simulink library "TYPEB_MASTER"  (Simulink 8.8)
settings: Solver=ode45  StartTime=0.0  StopTime=10.0  RelTol=1e-3  EnableMultiTasking=on
libraries: cdsEpicsOut x65, cdsTP x48, cdsFilt x34, cdsEpicsStringIn x29, cdsFiltCtrl x27, cdsRms x24, STATE_BIO_MASTER x15, cdsEpicsBinIn x14, cdsBit2Word x12, GAS_MASTER x9, cdsWord2Bit x5, cdsDacKill x4
(part 1 of 6)
settings Model: SuppressorTable=22 serialization::archive 11 0 3 0 0 0 11 0  Creator=controls  LastModifiedBy=controls

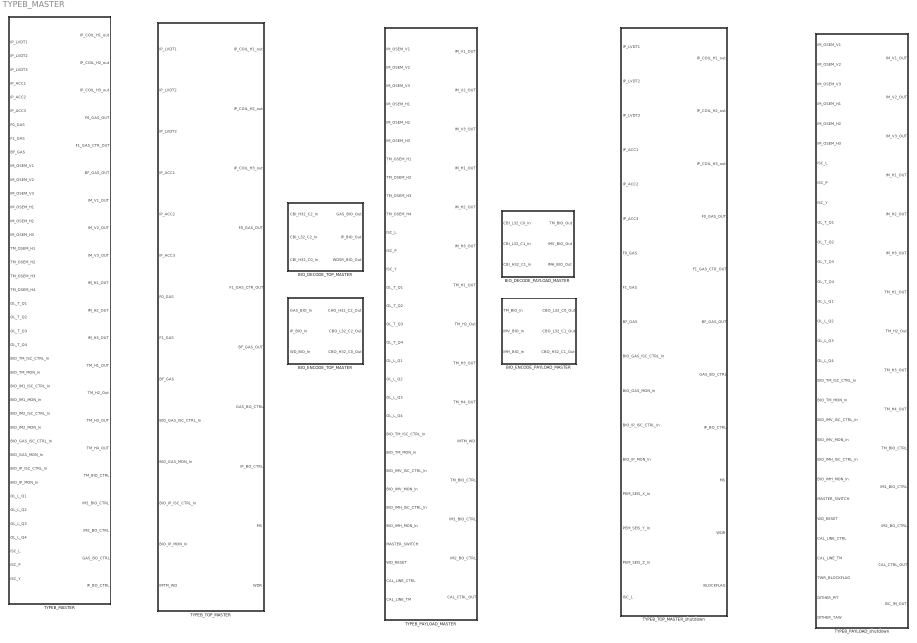
== system TYPEB_MASTER ==
  BIO_DECODE_PAYLOAD_MASTER : Subsystem
  BIO_DECODE_TOP_MASTER : Subsystem
  BIO_ENCODE_PAYLOAD_MASTER : Subsystem
  BIO_ENCODE_TOP_MASTER : Subsystem
  TYPEB_MASTER : Subsystem
  TYPEB_PAYLOAD_MASTER : Subsystem
  TYPEB_PAYLOAD_shutdown : Subsystem  AncestorBlock=TYPEB_MASTER/TYPEB_PAYLOAD_MASTER
  TYPEB_TOP_MASTER : Subsystem
  TYPEB_TOP_MASTER_shutdown : Subsystem  AncestorBlock=TYPEB_MASTER/TYPEB_TOP_MASTER

== system TYPEB_MASTER/BIO_DECODE_PAYLOAD_MASTER ==
  CBI_L32_C0_In : Inport
  CBI_L32_C1_In : Inport  Port=2
  CBI_H32_C1_In : Inport  Port=3
  BI0L_MON : cdsEpicsOut/Subsystem  Tag=cdsEpicsOutput  Description=|
      | Purpose:                                          
      | Output a FE signal to an EPICS channel.           
      |                                                   
      | Operation:                                        
      | Takes input value and passes it to EPICS record.  
      |                                                   
      | Usage:                                            
      | Name the part with the desired EPICS rrecord name.
      settings: AttributesFormatString=%<Tag>
  BI1H_MON : cdsEpicsOut/Subsystem  Tag=cdsEpicsOutput  Description=|
      | Purpose:                                          
      | Output a FE signal to an EPICS channel.           
      |                                                   
      | Operation:                                        
      | Takes input value and passes it to EPICS record.  
      |                                                   
      | Usage:                                            
      | Name the part with the desired EPICS rrecord name.
      settings: AttributesFormatString=%<Tag>
  BI1L_MON : cdsEpicsOut/Subsystem  Tag=cdsEpicsOutput  Description=|
      | Purpose:                                          
      | Output a FE signal to an EPICS channel.           
      |                                                   
      | Operation:                                        
      | Takes input value and passes it to EPICS record.  
      |                                                   
      | Usage:                                            
      | Name the part with the desired EPICS rrecord name.
      settings: AttributesFormatString=%<Tag>
  TM_BIO_Out : Outport
  IMV_BIO_Out : Outport  Port=2
  IMH_BIO_Out : Outport  Port=3
  wires:
  CBI_L32_C1_In/1 -> BI1L_MON/1
  CBI_L32_C0_In/1 -> BI0L_MON/1
  CBI_H32_C1_In/1 -> BI1H_MON/1
  BI0L_MON/1 -> TM_BIO_Out/1
  BI1L_MON/1 -> IMV_BIO_Out/1
  BI1H_MON/1 -> IMH_BIO_Out/1

== system TYPEB_MASTER/BIO_DECODE_TOP_MASTER ==
  CBI_H32_C2_In : Inport
  CBI_L32_C2_In : Inport  Port=2
  CBI_H32_C0_In : Inport  Port=3
  BI0H_MON : cdsEpicsOut/Subsystem  Tag=cdsEpicsOutput  Description=|
      | Purpose:                                          
      | Output a FE signal to an EPICS channel.           
      |                                                   
      | Operation:                                        
      | Takes input value and passes it to EPICS record.  
      |                                                   
      | Usage:                                            
      | Name the part with the desired EPICS rrecord name.
      settings: AttributesFormatString=%<Tag>
  BI2H_MON : cdsEpicsOut/Subsystem  Tag=cdsEpicsOutput  Description=|
      | Purpose:                                          
      | Output a FE signal to an EPICS channel.           
      |                                                   
      | Operation:                                        
      | Takes input value and passes it to EPICS record.  
      |                                                   
      | Usage:                                            
      | Name the part with the desired EPICS rrecord name.
      settings: AttributesFormatString=%<Tag>
  BI2L_MON : cdsEpicsOut/Subsystem  Tag=cdsEpicsOutput  Description=|
      | Purpose:                                          
      | Output a FE signal to an EPICS channel.           
      |                                                   
      | Operation:                                        
      | Takes input value and passes it to EPICS record.  
      |                                                   
      | Usage:                                            
      | Name the part with the desired EPICS rrecord name.
      settings: AttributesFormatString=%<Tag>
  GAS_BIO_Out : Outport
  IP_BIO_Out : Outport  Port=2
  WDSR_BIO_Out : Outport  Port=3
  wires:
  CBI_H32_C2_In/1 -> BI2H_MON/1
  CBI_L32_C2_In/1 -> BI2L_MON/1
  BI2H_MON/1 -> GAS_BIO_Out/1
  BI2L_MON/1 -> IP_BIO_Out/1
  CBI_H32_C0_In/1 -> BI0H_MON/1
  BI0H_MON/1 -> WDSR_BIO_Out/1

== system TYPEB_MASTER/BIO_ENCODE_PAYLOAD_MASTER ==
  TM_BIO_In : Inport
  IMV_BIO_In : Inport  Port=2
  IMH_BIO_In : Inport  Port=3
  BIT2WORD2 : Subsystem
  BIT2WORD3 : Subsystem
  BIT2WORD4 : Subsystem
  BO0L_OUT : cdsEpicsOut/Subsystem  Tag=cdsEpicsOutput  Description=|
      | Purpose:                                          
      | Output a FE signal to an EPICS channel.           
      |                                                   
      | Operation:                                        
      | Takes input value and passes it to EPICS record.  
      |                                                   
      | Usage:                                            
      | Name the part with the desired EPICS rrecord name.
      settings: AttributesFormatString=%<Tag>
  BO1H_OUT : cdsEpicsOut/Subsystem  Tag=cdsEpicsOutput  Description=|
      | Purpose:                                          
      | Output a FE signal to an EPICS channel.           
      |                                                   
      | Operation:                                        
      | Takes input value and passes it to EPICS record.  
      |                                                   
      | Usage:                                            
      | Name the part with the desired EPICS rrecord name.
      settings: AttributesFormatString=%<Tag>
  BO1L_OUT : cdsEpicsOut/Subsystem  Tag=cdsEpicsOutput  Description=|
      | Purpose:                                          
      | Output a FE signal to an EPICS channel.           
      |                                                   
      | Operation:                                        
      | Takes input value and passes it to EPICS record.  
      |                                                   
      | Usage:                                            
      | Name the part with the desired EPICS rrecord name.
      settings: AttributesFormatString=%<Tag>
  Ground{1..3,26,66..67} (6 alike) : Ground
  IMH_WD_RSET : cdsEpicsBinIn/Subsystem  Tag=cdsEpicsBinIn  Description=|
      | Purpose:                                                                            
      | Create an EPICS binary (0 or 1) input channel to the FE realtime controls.          
      |                                                                                     
      | Operation:                                                                          
      | Outputs value from an EPICS ai record. Value is binary input (bi Epics record type).
      |                                                                                     
      | Usage:                                                                              
      | Name the part with the desired EPICS channel name.
      settings: AttributesFormatString=%<Tag>
  IMV_WD_RSET : cdsEpicsBinIn/Subsystem  Tag=cdsEpicsBinIn  Description=|
      | Purpose:                                                                            
      | Create an EPICS binary (0 or 1) input channel to the FE realtime controls.          
      |                                                                                     
      | Operation:                                                                          
      | Outputs value from an EPICS ai record. Value is binary input (bi Epics record type).
      |                                                                                     
      | Usage:                                                                              
      | Name the part with the desired EPICS channel name.
      settings: AttributesFormatString=%<Tag>
  TM_WD_RSET : cdsEpicsBinIn/Subsystem  Tag=cdsEpicsBinIn  Description=|
      | Purpose:                                                                            
      | Create an EPICS binary (0 or 1) input channel to the FE realtime controls.          
      |                                                                                     
      | Operation:                                                                          
      | Outputs value from an EPICS ai record. Value is binary input (bi Epics record type).
      |                                                                                     
      | Usage:                                                                              
      | Name the part with the desired EPICS channel name.
      settings: AttributesFormatString=%<Tag>
  cdsWord2Bit : cdsWord2Bit/cdsWord2Bit  Tag=cdsWord2Bit  Description=Generate 16 0/1 outputs from single 16-bit integer input
      settings: AttributesFormatString=cdsWord2Bit
  cdsWord2Bit1 : cdsWord2Bit/cdsWord2Bit  Tag=cdsWord2Bit  Description=Generate 16 0/1 outputs from single 16-bit integer input
      settings: AttributesFormatString=cdsWord2Bit
  cdsWord2Bit2 : cdsWord2Bit/cdsWord2Bit  Tag=cdsWord2Bit  Description=Generate 16 0/1 outputs from single 16-bit integer input
      settings: AttributesFormatString=cdsWord2Bit
  CBO_L32_C0_Out : Outport
  CBO_L32_C1_Out : Outport  Port=2
  CBO_H32_C1_Out : Outport  Port=3
  wires:
  Ground2/1 -> BIT2WORD2/20(In20), BIT2WORD2/18(In18), BIT2WORD2/19(In19), BIT2WORD2/21(In21), BIT2WORD2/22(In22), BIT2WORD2/23(In23), BIT2WORD2/24(In24), BIT2WORD2/25(In25), BIT2WORD2/26(In26), BIT2WORD2/28(In28), BIT2WORD2/31(In31), BIT2WORD2/32(In32), BIT2WORD2/30(In30), BIT2WORD2/29(In29), BIT2WORD2/27(In27)
  TM_BIO_In/1 -> cdsWord2Bit/1
  cdsWord2Bit/4 -> BIT2WORD2/4(In4)
  cdsWord2Bit/5 -> BIT2WORD2/5(In5)
  cdsWord2Bit/3 -> BIT2WORD2/3(In3)
  cdsWord2Bit/2 -> BIT2WORD2/2(In2)
  cdsWord2Bit/6 -> BIT2WORD2/6(In6)
  cdsWord2Bit/1 -> BIT2WORD2/1(In1)
  cdsWord2Bit/7 -> BIT2WORD2/7(In7)
  cdsWord2Bit/8 -> BIT2WORD2/8(In8)
  cdsWord2Bit/9 -> BIT2WORD2/9(In9)
  cdsWord2Bit/10 -> BIT2WORD2/10(In10)
  cdsWord2Bit/11 -> BIT2WORD2/11(In11)
  Ground26/1 -> BIT2WORD3/20(In20), BIT2WORD3/18(In18), BIT2WORD3/19(In19), BIT2WORD3/21(In21), BIT2WORD3/22(In22), BIT2WORD3/23(In23), BIT2WORD3/24(In24), BIT2WORD3/25(In25), BIT2WORD3/26(In26), BIT2WORD3/28(In28), BIT2WORD3/31(In31), BIT2WORD3/32(In32), BIT2WORD3/30(In30), BIT2WORD3/29(In29), BIT2WORD3/27(In27)
  IMV_BIO_In/1 -> cdsWord2Bit1/1
  cdsWord2Bit1/4 -> BIT2WORD3/4(In4)
  cdsWord2Bit1/5 -> BIT2WORD3/5(In5)
  cdsWord2Bit1/3 -> BIT2WORD3/3(In3)
  cdsWord2Bit1/2 -> BIT2WORD3/2(In2)
  cdsWord2Bit1/6 -> BIT2WORD3/6(In6)
  cdsWord2Bit1/1 -> BIT2WORD3/1(In1)
  cdsWord2Bit1/7 -> BIT2WORD3/7(In7)
  cdsWord2Bit1/8 -> BIT2WORD3/8(In8)
  cdsWord2Bit1/9 -> BIT2WORD3/9(In9)
  cdsWord2Bit1/10 -> BIT2WORD3/10(In10)
  cdsWord2Bit1/11 -> BIT2WORD3/11(In11)
  Ground66/1 -> TM_WD_RSET/1
  Ground67/1 -> IMV_WD_RSET/1
  TM_WD_RSET/1 -> BIT2WORD2/17(In17)
  IMV_WD_RSET/1 -> BIT2WORD3/17(In17)
  BO0L_OUT/1 -> CBO_L32_C0_Out/1
  BO1H_OUT/1 -> CBO_H32_C1_Out/1
  BIT2WORD2/1(Out1) -> BO0L_OUT/1
  BIT2WORD3/1(Out1) -> BO1L_OUT/1
  BO1L_OUT/1 -> CBO_L32_C1_Out/1
  BIT2WORD4/1(Out1) -> BO1H_OUT/1
  Ground1/1 -> BIT2WORD4/27(In27), BIT2WORD4/26(In26), BIT2WORD4/25(In25), BIT2WORD4/24(In24), BIT2WORD4/23(In23), BIT2WORD4/22(In22), BIT2WORD4/21(In21), BIT2WORD4/20(In20), BIT2WORD4/19(In19), BIT2WORD4/18(In18), BIT2WORD4/28(In28), BIT2WORD4/29(In29), BIT2WORD4/30(In30), BIT2WORD4/32(In32), BIT2WORD4/31(In31)
  IMH_BIO_In/1 -> cdsWord2Bit2/1
  cdsWord2Bit2/4 -> BIT2WORD4/4(In4)
  cdsWord2Bit2/5 -> BIT2WORD4/5(In5)
  cdsWord2Bit2/3 -> BIT2WORD4/3(In3)
  cdsWord2Bit2/2 -> BIT2WORD4/2(In2)
  cdsWord2Bit2/6 -> BIT2WORD4/6(In6)
  cdsWord2Bit2/1 -> BIT2WORD4/1(In1)
  cdsWord2Bit2/7 -> BIT2WORD4/7(In7)
  cdsWord2Bit2/8 -> BIT2WORD4/8(In8)
  cdsWord2Bit2/9 -> BIT2WORD4/9(In9)
  cdsWord2Bit2/10 -> BIT2WORD4/10(In10)
  cdsWord2Bit2/11 -> BIT2WORD4/11(In11)
  Ground3/1 -> IMH_WD_RSET/1
  IMH_WD_RSET/1 -> BIT2WORD4/17(In17)
  cdsWord2Bit/12 -> BIT2WORD2/12(In12)
  cdsWord2Bit/13 -> BIT2WORD2/13(In13)
  cdsWord2Bit/14 -> BIT2WORD2/14(In14)
  cdsWord2Bit/15 -> BIT2WORD2/15(In15)
  cdsWord2Bit/16 -> BIT2WORD2/16(In16)
  cdsWord2Bit1/12 -> BIT2WORD3/12(In12)
  cdsWord2Bit1/16 -> BIT2WORD3/16(In16)
  cdsWord2Bit1/14 -> BIT2WORD3/14(In14)
  cdsWord2Bit1/15 -> BIT2WORD3/15(In15)
  cdsWord2Bit1/13 -> BIT2WORD3/13(In13)
  cdsWord2Bit2/13 -> BIT2WORD4/13(In13)
  cdsWord2Bit2/15 -> BIT2WORD4/15(In15)
  cdsWord2Bit2/14 -> BIT2WORD4/14(In14)
  cdsWord2Bit2/12 -> BIT2WORD4/12(In12)
  cdsWord2Bit2/16 -> BIT2WORD4/16(In16)

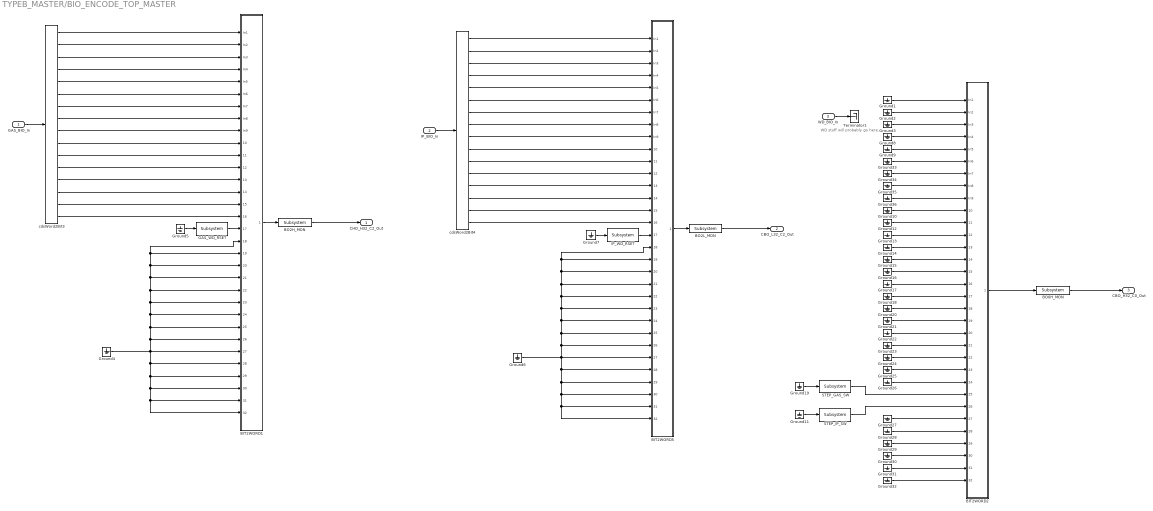
== system TYPEB_MASTER/BIO_ENCODE_TOP_MASTER ==
  note: WD stuff will probably go here.
  GAS_BIO_In : Inport
  IP_BIO_In : Inport  Port=2
  WD_BIO_In : Inport  Port=3
  BIT2WORD1 : Subsystem
  BIT2WORD2 : Subsystem
  BIT2WORD5 : Subsystem
  BO0H_MON : cdsEpicsOut/Subsystem  Tag=cdsEpicsOutput  Description=|
      | Purpose:                                          
      | Output a FE signal to an EPICS channel.           
      |                                                   
      | Operation:                                        
      | Takes input value and passes it to EPICS record.  
      |                                                   
      | Usage:                                            
      | Name the part with the desired EPICS rrecord name.
      settings: AttributesFormatString=%<Tag>
  BO2H_MON : cdsEpicsOut/Subsystem  Tag=cdsEpicsOutput  Description=|
      | Purpose:                                          
      | Output a FE signal to an EPICS channel.           
      |                                                   
      | Operation:                                        
      | Takes input value and passes it to EPICS record.  
      |                                                   
      | Usage:                                            
      | Name the part with the desired EPICS rrecord name.
      settings: AttributesFormatString=%<Tag>
  BO2L_MON : cdsEpicsOut/Subsystem  Tag=cdsEpicsOutput  Description=|
      | Purpose:                                          
      | Output a FE signal to an EPICS channel.           
      |                                                   
      | Operation:                                        
      | Takes input value and passes it to EPICS record.  
      |                                                   
      | Usage:                                            
      | Name the part with the desired EPICS rrecord name.
      settings: AttributesFormatString=%<Tag>
  GAS_WD_RSET : cdsEpicsBinIn/Subsystem  Tag=cdsEpicsBinIn  Description=|
      | Purpose:                                                                            
      | Create an EPICS binary (0 or 1) input channel to the FE realtime controls.          
      |                                                                                     
      | Operation:                                                                          
      | Outputs value from an EPICS ai record. Value is binary input (bi Epics record type).
      |                                                                                     
      | Usage:                                                                              
      | Name the part with the desired EPICS channel name.
      settings: AttributesFormatString=%<Tag>
  Ground{1..36} (36 alike) : Ground
  IP_WD_RSET : cdsEpicsBinIn/Subsystem  Tag=cdsEpicsBinIn  Description=|
      | Purpose:                                                                            
      | Create an EPICS binary (0 or 1) input channel to the FE realtime controls.          
      |                                                                                     
      | Operation:                                                                          
      | Outputs value from an EPICS ai record. Value is binary input (bi Epics record type).
      |                                                                                     
      | Usage:                                                                              
      | Name the part with the desired EPICS channel name.
      settings: AttributesFormatString=%<Tag>
  STEP_GAS_SW : cdsEpicsBinIn/Subsystem  Tag=cdsEpicsBinIn  Description=|
      | Purpose:                                                                            
      | Create an EPICS binary (0 or 1) input channel to the FE realtime controls.          
      |                                                                                     
      | Operation:                                                                          
      | Outputs value from an EPICS ai record. Value is binary input (bi Epics record type).
      |                                                                                     
      | Usage:                                                                              
      | Name the part with the desired EPICS channel name.
      settings: AttributesFormatString=%<Tag>
  STEP_IP_SW : cdsEpicsBinIn/Subsystem  Tag=cdsEpicsBinIn  Description=|
      | Purpose:                                                                            
      | Create an EPICS binary (0 or 1) input channel to the FE realtime controls.          
      |                                                                                     
      | Operation:                                                                          
      | Outputs value from an EPICS ai record. Value is binary input (bi Epics record type).
      |                                                                                     
      | Usage:                                                                              
      | Name the part with the desired EPICS channel name.
      settings: AttributesFormatString=%<Tag>
  Terminator1 : Terminator
  cdsWord2Bit3 : cdsWord2Bit/cdsWord2Bit  Tag=cdsWord2Bit  Description=Generate 16 0/1 outputs from single 16-bit integer input
      settings: AttributesFormatString=cdsWord2Bit
  cdsWord2Bit4 : cdsWord2Bit/cdsWord2Bit  Tag=cdsWord2Bit  Description=Generate 16 0/1 outputs from single 16-bit integer input
      settings: AttributesFormatString=cdsWord2Bit
  CHO_H32_C2_Out : Outport
  CBO_L32_C2_Out : Outport  Port=2
  CBO_H32_C0_Out : Outport  Port=3
  wires:
  BO0H_MON/1 -> CBO_H32_C0_Out/1
  BIT2WORD2/1(Out1) -> BO0H_MON/1
  BIT2WORD1/1(Out1) -> BO2H_MON/1
  BO2H_MON/1 -> CHO_H32_C2_Out/1
  Ground4/1 -> BIT2WORD1/27(In27), BIT2WORD1/26(In26), BIT2WORD1/25(In25), BIT2WORD1/24(In24), BIT2WORD1/23(In23), BIT2WORD1/22(In22), BIT2WORD1/21(In21), BIT2WORD1/20(In20), BIT2WORD1/19(In19), BIT2WORD1/18(In18), BIT2WORD1/28(In28), BIT2WORD1/29(In29), BIT2WORD1/30(In30), BIT2WORD1/32(In32), BIT2WORD1/31(In31)
  GAS_BIO_In/1 -> cdsWord2Bit3/1
  cdsWord2Bit3/4 -> BIT2WORD1/4(In4)
  cdsWord2Bit3/5 -> BIT2WORD1/5(In5)
  cdsWord2Bit3/3 -> BIT2WORD1/3(In3)
  cdsWord2Bit3/2 -> BIT2WORD1/2(In2)
  cdsWord2Bit3/6 -> BIT2WORD1/6(In6)
  cdsWord2Bit3/1 -> BIT2WORD1/1(In1)
  cdsWord2Bit3/7 -> BIT2WORD1/7(In7)
  cdsWord2Bit3/8 -> BIT2WORD1/8(In8)
  cdsWord2Bit3/9 -> BIT2WORD1/9(In9)
  cdsWord2Bit3/10 -> BIT2WORD1/10(In10)
  cdsWord2Bit3/11 -> BIT2WORD1/11(In11)
  Ground5/1 -> GAS_WD_RSET/1
  GAS_WD_RSET/1 -> BIT2WORD1/17(In17)
  cdsWord2Bit3/13 -> BIT2WORD1/13(In13)
  cdsWord2Bit3/14 -> BIT2WORD1/14(In14)
  cdsWord2Bit3/15 -> BIT2WORD1/15(In15)
  cdsWord2Bit3/16 -> BIT2WORD1/16(In16)
  cdsWord2Bit3/12 -> BIT2WORD1/12(In12)
  BIT2WORD5/1(Out1) -> BO2L_MON/1
  BO2L_MON/1 -> CBO_L32_C2_Out/1
  Ground6/1 -> BIT2WORD5/27(In27), BIT2WORD5/26(In26), BIT2WORD5/25(In25), BIT2WORD5/24(In24), BIT2WORD5/23(In23), BIT2WORD5/22(In22), BIT2WORD5/21(In21), BIT2WORD5/20(In20), BIT2WORD5/19(In19), BIT2WORD5/18(In18), BIT2WORD5/28(In28), BIT2WORD5/29(In29), BIT2WORD5/30(In30), BIT2WORD5/32(In32), BIT2WORD5/31(In31)
  IP_BIO_In/1 -> cdsWord2Bit4/1
  cdsWord2Bit4/4 -> BIT2WORD5/4(In4)
  cdsWord2Bit4/5 -> BIT2WORD5/5(In5)
  cdsWord2Bit4/3 -> BIT2WORD5/3(In3)
  cdsWord2Bit4/2 -> BIT2WORD5/2(In2)
  cdsWord2Bit4/6 -> BIT2WORD5/6(In6)
  cdsWord2Bit4/1 -> BIT2WORD5/1(In1)
  cdsWord2Bit4/7 -> BIT2WORD5/7(In7)
  cdsWord2Bit4/8 -> BIT2WORD5/8(In8)
  cdsWord2Bit4/9 -> BIT2WORD5/9(In9)
  cdsWord2Bit4/10 -> BIT2WORD5/10(In10)
  cdsWord2Bit4/11 -> BIT2WORD5/11(In11)
  Ground7/1 -> IP_WD_RSET/1
  IP_WD_RSET/1 -> BIT2WORD5/17(In17)
  cdsWord2Bit4/13 -> BIT2WORD5/13(In13)
  cdsWord2Bit4/14 -> BIT2WORD5/14(In14)
  cdsWord2Bit4/15 -> BIT2WORD5/15(In15)
  cdsWord2Bit4/16 -> BIT2WORD5/16(In16)
  cdsWord2Bit4/12 -> BIT2WORD5/12(In12)
  Ground29/1 -> BIT2WORD2/29(In29)
  Ground30/1 -> BIT2WORD2/30(In30)
  Ground32/1 -> BIT2WORD2/32(In32)
  Ground27/1 -> BIT2WORD2/27(In27)
  Ground31/1 -> BIT2WORD2/31(In31)
  Ground28/1 -> BIT2WORD2/28(In28)
  Ground23/1 -> BIT2WORD2/21(In21)
  Ground25/1 -> BIT2WORD2/23(In23)
  Ground26/1 -> BIT2WORD2/24(In24)
  Ground24/1 -> BIT2WORD2/22(In22)
  Ground21/1 -> BIT2WORD2/19(In19)
  Ground18/1 -> BIT2WORD2/17(In17)
  Ground22/1 -> BIT2WORD2/20(In20)
  Ground20/1 -> BIT2WORD2/18(In18)
  Ground3/1 -> BIT2WORD2/3(In3)
  Ground17/1 -> BIT2WORD2/16(In16)
  Ground16/1 -> BIT2WORD2/15(In15)
  Ground10/1 -> BIT2WORD2/10(In10)
  Ground15/1 -> BIT2WORD2/14(In14)
  Ground34/1 -> BIT2WORD2/7(In7)
  Ground8/1 -> BIT2WORD2/4(In4)
  Ground13/1 -> BIT2WORD2/12(In12)
  Ground35/1 -> BIT2WORD2/8(In8)
  Ground1/1 -> BIT2WORD2/1(In1)
  Ground33/1 -> BIT2WORD2/6(In6)
  Ground36/1 -> BIT2WORD2/9(In9)
  Ground2/1 -> BIT2WORD2/2(In2)
  Ground14/1 -> BIT2WORD2/13(In13)
  Ground12/1 -> BIT2WORD2/11(In11)
  Ground9/1 -> BIT2WORD2/5(In5)
  Ground11/1 -> STEP_IP_SW/1
  Ground19/1 -> STEP_GAS_SW/1
  STEP_IP_SW/1 -> BIT2WORD2/26(In26)
  STEP_GAS_SW/1 -> BIT2WORD2/25(In25)
  WD_BIO_In/1 -> Terminator1/1

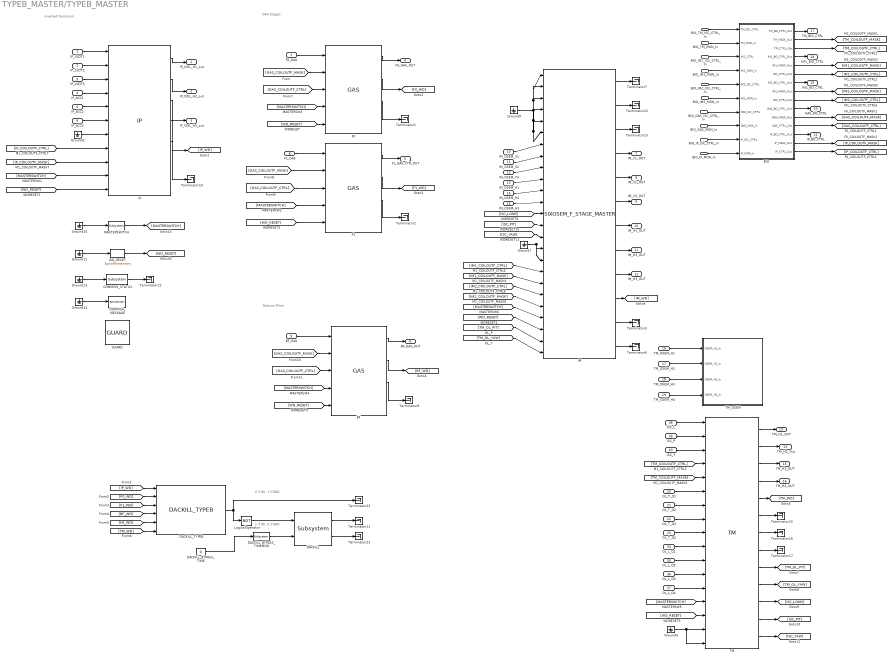
== system TYPEB_MASTER/TYPEB_MASTER ==
  note: GAS Stages
  note: Bottom Filter
  note: Inverted Pendulum
  note: 0 if OK, 1 if BAD
  note: 1 if OK, 0 if BAD
  IP_LVDT1 : Inport
  IP_LVDT2 : Inport  Port=2
  IP_LVDT3 : Inport  Port=3
  IP_ACC1 : Inport  Port=4
  IP_ACC2 : Inport  Port=5
  IP_ACC3 : Inport  Port=6
  F0_GAS : Inport  Port=7
  F1_GAS : Inport  Port=8
  BF_GAS : Inport  Port=9
  IM_OSEM_V1 : Inport  Port=10
  IM_OSEM_V2 : Inport  Port=11
  IM_OSEM_V3 : Inport  Port=12
  IM_OSEM_H1 : Inport  Port=13
  IM_OSEM_H2 : Inport  Port=14
  IM_OSEM_H3 : Inport  Port=15
  TM_OSEM_H1 : Inport  Port=16
  TM_OSEM_H2 : Inport  Port=17
  TM_OSEM_H3 : Inport  Port=18
  TM_OSEM_H4 : Inport  Port=19
  OL_T_Q1 : Inport  Port=20
  OL_T_Q2 : Inport  Port=21
  OL_T_Q3 : Inport  Port=22
  OL_T_Q4 : Inport  Port=23
  BIO_TM_ISC_CTRL_In : Inport  Port=24
  BIO_TM_MON_In : Inport  Port=25
  BIO_IM1_ISC_CTRL_In : Inport  Port=26
  BIO_IM1_MON_In : Inport  Port=27
  BIO_IM2_ISC_CTRL_In : Inport  Port=28
  BIO_IM2_MON_In : Inport  Port=29
  BIO_GAS_ISC_CTRL_In : Inport  Port=30
  BIO_GAS_MON_In : Inport  Port=31
  BIO_IP_ISC_CTRL_In : Inport  Port=32
  BIO_IP_MON_In : Inport  Port=33
  OL_L_Q1 : Inport  Port=34
  OL_L_Q2 : Inport  Port=35
  OL_L_Q3 : Inport  Port=36
  OL_L_Q4 : Inport  Port=37
  ISC_L : Inport  Port=38
  ISC_P : Inport  Port=39
  ISC_Y : Inport  Port=40
  BF : GAS_MASTER/GAS
  BIO : Subsystem
  COMMISH_MESSAGE : cdsEpicsStringIn/EpicsStringIn  Tag=cdsEpicsStringIn  Description=cdsEpicsStringIn
      settings: AttributesFormatString=%<Tag>
  COMMISH_STATUS : cdsEpicsBinIn/Subsystem  Tag=cdsEpicsBinIn  Description=|
      | Purpose:                                                                            
      | Create an EPICS binary (0 or 1) input channel to the FE realtime controls.          
      |                                                                                     
      | Operation:                                                                          
      | Outputs value from an EPICS ai record. Value is binary input (bi Epics record type).
      |                                                                                     
      | Usage:                                                                              
      | Name the part with the desired EPICS channel name.
      settings: AttributesFormatString=%<Tag>
  DACKILL : cdsDacKill/Subsystem  Description=cdsDacKill
      settings: AttributesFormatString=%<Description>
  DACKILL_BYPASS_TIME : Constant  Value=0
  DACKILL_BYPASS_TIMEMON : cdsEpicsOut/Subsystem  Tag=cdsEpicsOutput  Description=|
      | Purpose:                                          
      | Output a FE signal to an EPICS channel.           
      |                                                   
      | Operation:                                        
      | Takes input value and passes it to EPICS record.  
      |                                                   
      | Usage:                                            
      | Name the part with the desired EPICS rrecord name.
      settings: AttributesFormatString=%<Tag>
  DACKILL_TYPEB : VIS_LIB/DACKILL_TYPEB
  F0 : GAS_MASTER/GAS
  F1 : GAS_MASTER/GAS
  GUARD : ISC_common/GUARD
  Ground{3,5,7,9..11,13..14} (8 alike) : Ground
  IM : SIXOSEM_F_STAGE_MASTER/SIXOSEM_F_STAGE_MASTER  Description=SIXOSEMSTAGE_FACE_MASTER
  IP : IP_MASTER/IP
  LogicalOperator : Logic  Operator=NOT  AllPortsSameDT=off  OutDataTypeStr=boolean
  MASTERSWITCH : cdsEpicsBinIn/Subsystem  Tag=cdsEpicsBinIn  Description=|
      | Purpose:                                                                            
      | Create an EPICS binary (0 or 1) input channel to the FE realtime controls.          
      |                                                                                     
      | Operation:                                                                          
      | Outputs value from an EPICS ai record. Value is binary input (bi Epics record type).
      |                                                                                     
      | Usage:                                                                              
      | Name the part with the desired EPICS channel name.
      settings: AttributesFormatString=%<Tag>
  TM : TM_MASTER/TM
  TM_OSEM : Subsystem
  Terminator{1..2,5..7,9..13,15..17,21..23} (16 alike) : Terminator
  WD_RESET : cdsEpicsMomentary/EpicsMomentary  Tag=cdsEpicsMomentary
      settings: AttributesFormatString=%<Tag>
  IP_COIL_H1_out : Outport
  IP_COIL_H2_out : Outport  Port=2
  IP_COIL_H3_out : Outport  Port=3
  F0_GAS_OUT : Outport  Port=4
  F1_GAS_CTR_OUT : Outport  Port=5
  BF_GAS_OUT : Outport  Port=6
  IM_V1_OUT : Outport  Port=7
  IM_V2_OUT : Outport  Port=8
  IM_V3_OUT : Outport  Port=9
  IM_H1_OUT : Outport  Port=10
  IM_H2_OUT : Outport  Port=11
  IM_H3_OUT : Outport  Port=12
  TM_H1_OUT : Outport  Port=13
  TM_H2_Out : Outport  Port=14
  TM_H3_OUT : Outport  Port=15
  TM_H4_OUT : Outport  Port=16
  TM_BIO_CTRL : Outport  Port=17
  IM1_BIO_CTRL : Outport  Port=18
  IM2_BO_CTRL : Outport  Port=19
  GAS_BO_CTRL : Outport  Port=20
  IP_BO_CTRL : Outport  Port=21
  wires:
  F0/2 -> [F0_WD]
  F0/3 -> Terminator1/1
  F1/3 -> Terminator2/1
  F1/2 -> [F1_WD]
  BF/1 -> BF_GAS_OUT/1
  Ground3/1 -> IP/7
  IP_LVDT2/1 -> IP/2
  IP_LVDT1/1 -> IP/1
  IP_ACC2/1 -> IP/5
  IP_LVDT3/1 -> IP/3
  IP_ACC1/1 -> IP/4
  IP_ACC3/1 -> IP/6
  F0_GAS/1 -> F0/1
  F1_GAS/1 -> F1/1
  BF_GAS/1 -> BF/1
  F0/1 -> F0_GAS_OUT/1
  F1/1 -> F1_GAS_CTR_OUT/1
  IP/1 -> IP_COIL_H1_out/1
  IP/2 -> IP_COIL_H2_out/1
  IP/3 -> IP_COIL_H3_out/1
  IP/4 -> [IP_WD]
  IP/5 -> Terminator10/1
  IM/10 -> [IM_WD]
  IM/11 -> Terminator5/1
  IM/12 -> Terminator6/1
  IM/1 -> Terminator7/1
  IM/2 -> Terminator12/1
  IM/3 -> Terminator13/1
  TM/5 -> [TM_WD]
  TM/6 -> Terminator15/1
  TM/7 -> Terminator16/1
  TM/8 -> Terminator17/1
  Ground5/1 -> TM/17, TM/16
  TM_OSEM_H3/1 -> TM_OSEM/3(OSEM_H3_In)
  TM_OSEM_H2/1 -> TM_OSEM/2(OSEM_H2_In)
  TM_OSEM_H4/1 -> TM_OSEM/4(OSEM_H4_In)
  TM_OSEM_H1/1 -> TM_OSEM/1(OSEM_H1_In)
  OL_T_Q4/1 -> TM/9
  OL_T_Q3/1 -> TM/8
  OL_T_Q1/1 -> TM/6
  OL_T_Q2/1 -> TM/7
  Ground10/1 -> MASTERSWITCH/1
  MASTERSWITCH/1 -> [MASTERSWITCH]
  [MASTERSWITCH] -> BF/4
  [MASTERSWITCH] -> TM/14
  WD_RESET/1 -> [WD_RESET]
  Ground11/1 -> WD_RESET/1
  [WD_RESET] -> F0/5
  [WD_RESET] -> F1/5
  [WD_RESET] -> BF/5
  [WD_RESET] -> TM/15
  [GAS_COILOUTF_CTRL] -> F1/3
  Ground14/1 -> COMMISH_MESSAGE/1
  COMMISH_STATUS/1 -> Terminator21/1
  Ground13/1 -> COMMISH_STATUS/1
  [MASTERSWITCH] -> F1/4
  [GAS_COILOUTF_MASK] -> F1/2
  [MASTERSWITCH] -> F0/4
  [IP_WD] -> DACKILL_TYPEB/1
  DACKILL_TYPEB/1 -> Terminator23/1, LogicalOperator/1
  LogicalOperator/1 -> DACKILL/1
  DACKILL_BYPASS_TIMEMON/1 -> DACKILL/2
  DACKILL_BYPASS_TIME/1 -> DACKILL_BYPASS_TIMEMON/1
  DACKILL/1 -> Terminator11/1
  DACKILL/2 -> Terminator22/1
  [F0_WD] -> DACKILL_TYPEB/2
  [F1_WD] -> DACKILL_TYPEB/3
  [TM_WD] -> DACKILL_TYPEB/6
  [BF_WD] -> DACKILL_TYPEB/4
  [IM_WD] -> DACKILL_TYPEB/5
  [TM_COILOUTF_CTRL] -> TM/4
  [TM_COILOUTF_MASK] -> TM/5
  BF/2 -> [BF_WD]
  BF/3 -> Terminator9/1
  IM/4 -> IM_V1_OUT/1
  IM/5 -> IM_V2_OUT/1
  IM/6 -> IM_V3_OUT/1
  IM/7 -> IM_H1_OUT/1
  IM/8 -> IM_H2_OUT/1
  IM/9 -> IM_H3_OUT/1
  TM/1 -> TM_H1_OUT/1
  TM/2 -> TM_H2_Out/1
  TM/3 -> TM_H3_OUT/1
  TM/4 -> TM_H4_OUT/1
  Ground9/1 -> IM/6, IM/5, IM/4, IM/1, IM/2, IM/3
  IM_OSEM_V1/1 -> IM/7
  IM_OSEM_V2/1 -> IM/8
  IM_OSEM_V3/1 -> IM/9
  IM_OSEM_H1/1 -> IM/10
  IM_OSEM_H2/1 -> IM/11
  IM_OSEM_H3/1 -> IM/12
  [IM1_COILOUTF_CTRL] -> IM/18
  [IM1_COILOUTF_MASK] -> IM/19
  BIO_TM_ISC_CTRL_In/1 -> BIO/1(TM_ISC_CTRL)
  BIO_TM_MON_In/1 -> BIO/2(TM_MON_In)
  BIO_IM1_ISC_CTRL_In/1 -> BIO/3(IM1_CTRL)
  BIO_IM1_MON_In/1 -> BIO/4(IM1_MON_In)
  BIO_IM2_ISC_CTRL_In/1 -> BIO/5(IM2_ISC_CTRL)
  BIO_IM2_MON_In/1 -> BIO/6(IM2_MON_In)
  BIO_GAS_ISC_CTRL_In/1 -> BIO/7(GAS_ISC_CTRL)
  BIO_GAS_MON_In/1 -> BIO/8(GAS_MON_In)
  BIO_IP_ISC_CTRL_In/1 -> BIO/9(IP_ISC_CTRL)
  BIO_IP_MON_In/1 -> BIO/10(IP_MON_In)
  BIO/1(TM_BO_CTRL_Out) -> TM_BIO_CTRL/1
  BIO/4(IM1_BO_CTRL_Out) -> IM1_BIO_CTRL/1
  BIO/7(IM2_BO_CTRL_Out) -> IM2_BO_CTRL/1
  BIO/10(GAS_BO_CTRL_Out) -> GAS_BO_CTRL/1
  BIO/13(IP_BO_CTRL_Out) -> IP_BO_CTRL/1
  BIO/5(IM1_MASK_Out) -> [IM1_COILOUTF_MASK]
  BIO/6(IM1_CTRL_Out) -> [IM1_COILOUTF_CTRL]
  BIO/2(TM_MASK_Out) -> [TM_COILOUTF_MASK]
  BIO/3(TM_CTRL_Out) -> [TM_COILOUTF_CTRL]
  BIO/8(IM2_MASK_Out) -> [IM2_COILOUTF_MASK]
  BIO/9(IM2_CTRL_Out) -> [IM2_COILOUTF_CTRL]
  BIO/11(GAS_MASK_Out) -> [GAS_COILOUTF_MASK]
  BIO/12(GAS_CTRL_Out) -> [GAS_COILOUTF_CTRL]
  BIO/14(IP_MASK_Out) -> [IP_COILOUTF_MASK]
  BIO/15(IP_CTRL_Out) -> [IP_COILOUTF_CTRL]
  OL_L_Q4/1 -> TM/13
  OL_L_Q3/1 -> TM/12
  OL_L_Q1/1 -> TM/10
  OL_L_Q2/1 -> TM/11
  [WD_RESET] -> IM/23
  [MASTERSWITCH] -> IM/22
  TM/10 -> [TM_OL_YAW]
  TM/9 -> [TM_OL_PIT]
  [TM_OL_YAW] -> IM/25
  [TM_OL_PIT] -> IM/24
  [WD_RESET] -> IP/11
  [MASTERSWITCH] -> IP/10
  [IM2_COILOUTF_CTRL] -> IM/20
  [IM2_COILOUTF_MASK] -> IM/21
  [IP_COILOUTF_CTRL] -> IP/8
  [IP_COILOUTF_MASK] -> IP/9
  [GAS_COILOUTF_MASK] -> F0/2
  [GAS_COILOUTF_CTRL] -> F0/3
  [GAS_COILOUTF_MASK] -> BF/2
  [GAS_COILOUTF_CTRL] -> BF/3
  [ISC_LONG] -> IM/13
  [ISC_PIT] -> IM/14
  [ISC_YAW] -> IM/15
  Ground7/1 -> IM/17, IM/16
  ISC_Y/1 -> TM/3
  ISC_L/1 -> TM/1
  ISC_P/1 -> TM/2
  TM/11 -> [ISC_LONG]
  TM/12 -> [ISC_PIT]
  TM/13 -> [ISC_YAW]

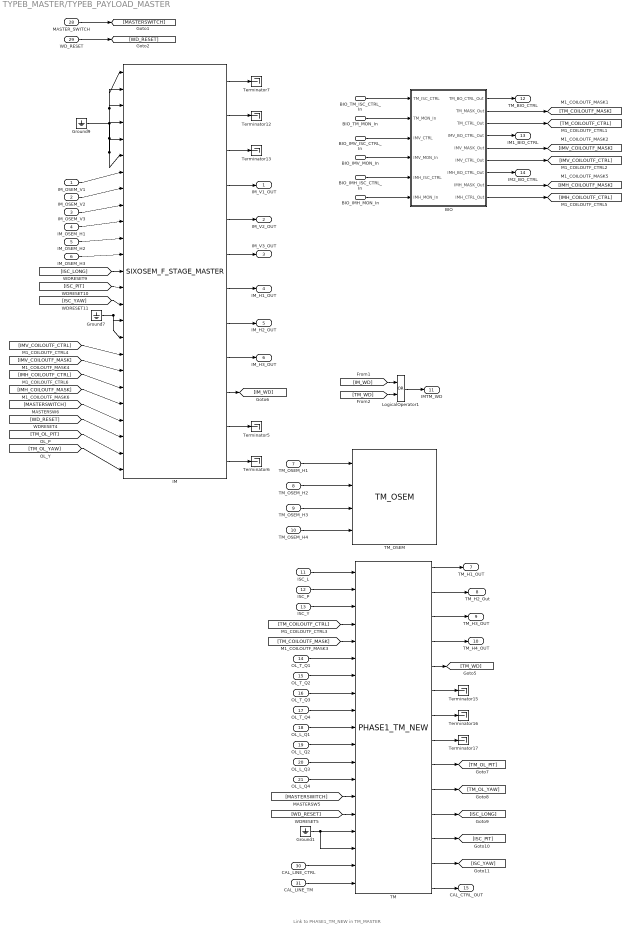
== system TYPEB_MASTER/TYPEB_PAYLOAD_MASTER ==
  note: Link to PHASE1_TM_NEW in TM_MASTER
  IM_OSEM_V1 : Inport
  IM_OSEM_V2 : Inport  Port=2
  IM_OSEM_V3 : Inport  Port=3
  IM_OSEM_H1 : Inport  Port=4
  IM_OSEM_H2 : Inport  Port=5
  IM_OSEM_H3 : Inport  Port=6
  TM_OSEM_H1 : Inport  Port=7
  TM_OSEM_H2 : Inport  Port=8
  TM_OSEM_H3 : Inport  Port=9
  TM_OSEM_H4 : Inport  Port=10
  ISC_L : Inport  Port=11
  ISC_P : Inport  Port=12
  ISC_Y : Inport  Port=13
  OL_T_Q1 : Inport  Port=14
  OL_T_Q2 : Inport  Port=15
  OL_T_Q3 : Inport  Port=16
  OL_T_Q4 : Inport  Port=17
  OL_L_Q1 : Inport  Port=18
  OL_L_Q2 : Inport  Port=19
  OL_L_Q3 : Inport  Port=20
  OL_L_Q4 : Inport  Port=21
  BIO_TM_ISC_CTRL_In : Inport  Port=22
  BIO_TM_MON_In : Inport  Port=23
  BIO_IMV_ISC_CTRL_In : Inport  Port=24
  BIO_IMV_MON_In : Inport  Port=25
  BIO_IMH_ISC_CTRL_In : Inport  Port=26
  BIO_IMH_MON_In : Inport  Port=27
  MASTER_SWITCH : Inport  Port=28
  WD_RESET : Inport  Port=29
  CAL_LINE_CTRL : Inport  Port=30
  CAL_LINE_TM : Inport  Port=31
  BIO : Subsystem
  Ground1 : Ground
  Ground7 : Ground
  Ground9 : Ground
  IM : SIXOSEM_F_STAGE_MASTER/SIXOSEM_F_STAGE_MASTER  Description=SIXOSEMSTAGE_FACE_MASTER
  LogicalOperator1 : Logic  Operator=OR  AllPortsSameDT=off  OutDataTypeStr=boolean
  TM : TM_MASTER/PHASE1_TM_NEW
  TM_OSEM : TYPEB_MASTER/TYPEB_MASTER/TM_OSEM
  Terminator{5..7,12..13,15..17} (8 alike) : Terminator
  IM_V1_OUT : Outport
  IM_V2_OUT : Outport  Port=2
  IM_V3_OUT : Outport  Port=3
  IM_H1_OUT : Outport  Port=4
  IM_H2_OUT : Outport  Port=5
  IM_H3_OUT : Outport  Port=6
  TM_H1_OUT : Outport  Port=7
  TM_H2_Out : Outport  Port=8
  TM_H3_OUT : Outport  Port=9
  TM_H4_OUT : Outport  Port=10
  IMTM_WD : Outport  Port=11
  TM_BIO_CTRL : Outport  Port=12
  IM1_BIO_CTRL : Outport  Port=13
  IM2_BO_CTRL : Outport  Port=14
  CAL_CTRL_OUT : Outport  Port=15
  wires:
  IM/1 -> Terminator7/1
  IM/12 -> Terminator6/1
  IM/5 -> IM_V2_OUT/1
  IM/6 -> IM_V3_OUT/1
  IM/7 -> IM_H1_OUT/1
  IM/8 -> IM_H2_OUT/1
  IM/9 -> IM_H3_OUT/1
  TM/1 -> TM_H1_OUT/1
  TM/3 -> TM_H3_OUT/1
  TM/2 -> TM_H2_Out/1
  Ground9/1 -> IM/6, IM/5, IM/4, IM/1, IM/2, IM/3
  TM/4 -> TM_H4_OUT/1
  IM_OSEM_V2/1 -> IM/8
  IM_OSEM_V1/1 -> IM/7
  IM_OSEM_H1/1 -> IM/10
  IM_OSEM_V3/1 -> IM/9
  IM_OSEM_H3/1 -> IM/12
  IM_OSEM_H2/1 -> IM/11
  [IMV_COILOUTF_MASK] -> IM/19
  IM/2 -> Terminator12/1
  TM/7 -> Terminator16/1
  TM/6 -> Terminator15/1
  Ground1/1 -> TM/17, TM/16
  TM/8 -> Terminator17/1
  TM_OSEM_H3/1 -> TM_OSEM/3
  TM_OSEM_H2/1 -> TM_OSEM/2
  TM_OSEM_H4/1 -> TM_OSEM/4
  OL_T_Q4/1 -> TM/9
  TM_OSEM_H1/1 -> TM_OSEM/1
  OL_T_Q1/1 -> TM/6
  OL_T_Q3/1 -> TM/8
  [MASTERSWITCH] -> TM/14
  OL_T_Q2/1 -> TM/7
  [TM_COILOUTF_CTRL] -> TM/4
  [WD_RESET] -> TM/15
  [TM_COILOUTF_MASK] -> TM/5
  IM/4 -> IM_V1_OUT/1
  IM/3 -> Terminator13/1
  TM/5 -> [TM_WD]
  IM/10 -> [IM_WD]
  TM/13 -> [ISC_YAW]
  [IMV_COILOUTF_CTRL] -> IM/18
  OL_L_Q3/1 -> TM/12
  OL_L_Q4/1 -> TM/13
  OL_L_Q2/1 -> TM/11
  OL_L_Q1/1 -> TM/10
  [WD_RESET] -> IM/23
  [MASTERSWITCH] -> IM/22
  TM/10 -> [TM_OL_YAW]
  TM/9 -> [TM_OL_PIT]
  [TM_OL_PIT] -> IM/24
  [TM_OL_YAW] -> IM/25
  [IMH_COILOUTF_MASK] -> IM/21
  [IMH_COILOUTF_CTRL] -> IM/20
  [ISC_LONG] -> IM/13
  [ISC_PIT] -> IM/14
  [ISC_YAW] -> IM/15
  Ground7/1 -> IM/17, IM/16
  ISC_Y/1 -> TM/3
  ISC_L/1 -> TM/1
  ISC_P/1 -> TM/2
  TM/11 -> [ISC_LONG]
  TM/12 -> [ISC_PIT]
  IM/11 -> Terminator5/1
  [IM_WD] -> LogicalOperator1/1
  [TM_WD] -> LogicalOperator1/2
  LogicalOperator1/1 -> IMTM_WD/1
  BIO/8(IMH_MASK_Out) -> [IMH_COILOUTF_MASK]
  BIO_TM_MON_In/1 -> BIO/2(TM_MON_In)
  BIO/4(IMV_BO_CTRL_Out) -> IM1_BIO_CTRL/1
  BIO_TM_ISC_CTRL_In/1 -> BIO/1(TM_ISC_CTRL)
  BIO_IMV_ISC_CTRL_In/1 -> BIO/3(IMV_CTRL)
  BIO_IMV_MON_In/1 -> BIO/4(IMV_MON_In)
  BIO/1(TM_BO_CTRL_Out) -> TM_BIO_CTRL/1
  BIO/7(IMH_BO_CTRL_Out) -> IM2_BO_CTRL/1
  BIO/5(IMV_MASK_Out) -> [IMV_COILOUTF_MASK]
  BIO/6(IMV_CTRL_Out) -> [IMV_COILOUTF_CTRL]
  BIO/2(TM_MASK_Out) -> [TM_COILOUTF_MASK]
  BIO/3(TM_CTRL_Out) -> [TM_COILOUTF_CTRL]
  BIO/9(IMH_CTRL_Out) -> [IMH_COILOUTF_CTRL]
  BIO_IMH_ISC_CTRL_In/1 -> BIO/5(IMH_ISC_CTRL)
  BIO_IMH_MON_In/1 -> BIO/6(IMH_MON_In)
  MASTER_SWITCH/1 -> [MASTERSWITCH]
  WD_RESET/1 -> [WD_RESET]
  CAL_LINE_CTRL/1 -> TM/18
  CAL_LINE_TM/1 -> TM/19
  TM/14 -> CAL_CTRL_OUT/1

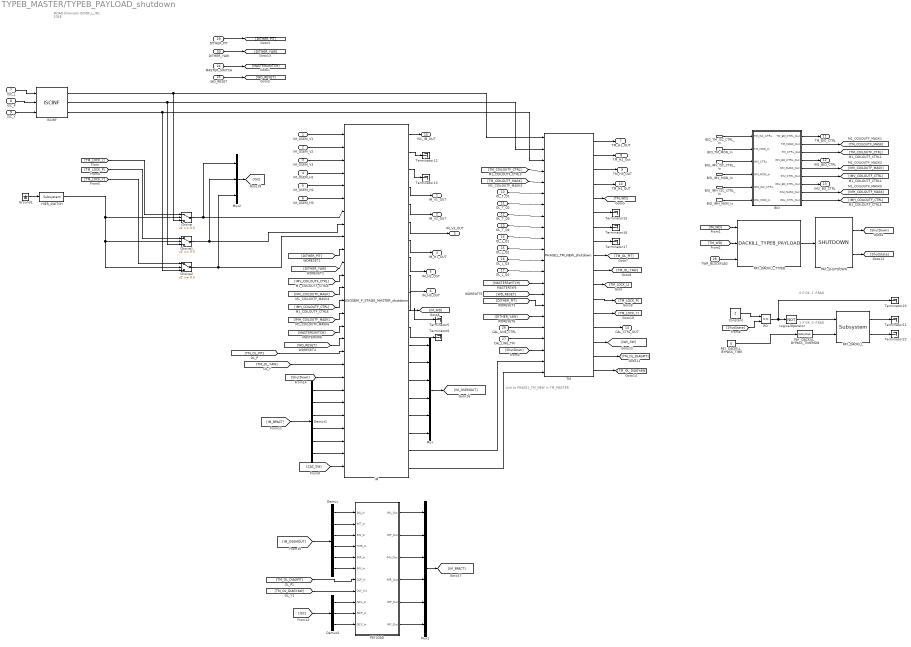
== system TYPEB_MASTER/TYPEB_PAYLOAD_shutdown ==
  note: Link to PHASE1_TM_NEW in TM_MASTER
  note: 0 if OK, 1 if BAD
  note: 1 if OK, 0 if BAD
  note: #DAQ Channels
      | ISCINF_L_IN1 2048
  IM_OSEM_V1 : Inport
  IM_OSEM_V2 : Inport  Port=2
  IM_OSEM_V3 : Inport  Port=3
  IM_OSEM_H1 : Inport  Port=4
  IM_OSEM_H2 : Inport  Port=5
  IM_OSEM_H3 : Inport  Port=6
  ISC_L : Inport  Port=7
  ISC_P : Inport  Port=8
  ISC_Y : Inport  Port=9
  OL_T_Q1 : Inport  Port=10
  OL_T_Q2 : Inport  Port=11
  OL_T_Q3 : Inport  Port=12
  OL_T_Q4 : Inport  Port=13
  OL_L_Q1 : Inport  Port=14
  OL_L_Q2 : Inport  Port=15
  OL_L_Q3 : Inport  Port=16
  OL_L_Q4 : Inport  Port=17
  BIO_TM_ISC_CTRL_In : Inport  Port=18
  BIO_TM_MON_In : Inport  Port=19
  BIO_IMV_ISC_CTRL_In : Inport  Port=20
  BIO_IMV_MON_In : Inport  Port=21
  BIO_IMH_ISC_CTRL_In : Inport  Port=22
  BIO_IMH_MON_In : Inport  Port=23
  MASTER_SWITCH : Inport  Port=24
  WD_RESET : Inport  Port=25
  CAL_LINE_CTRL : Inport  Port=26
  CAL_LINE_TM : Inport  Port=27
  TWR_BLOCKFLAG : Inport  Port=28
  DITHER_PIT : Inport  Port=29
  DITHER_YAW : Inport  Port=30
  BIO : Subsystem
  Choice : Switch  Threshold=0.5
  Choice1 : Switch  Threshold=0.5
  Choice2 : Switch  Threshold=0.5
  Constant : Constant  Value=2
  Demux : Demux  Outputs=6
  Demux1 : Demux  Outputs=6
  Demux2 : Demux  Outputs=3
  Ground1 : Ground
  HIER_SWITCH : cdsEpicsBinIn/Subsystem  Tag=cdsEpicsBinIn  Description=|
      | Purpose:                                                                            
      | Create an EPICS binary (0 or 1) input channel to the FE realtime controls.          
      |                                                                                     
      | Operation:                                                                          
      | Outputs value from an EPICS ai record. Value is binary input (bi Epics record type).
      |                                                                                     
      | Usage:                                                                              
      | Name the part with the desired EPICS channel name.
      settings: AttributesFormatString=%<Tag>
  IM : SIXOSEM_F_STAGE_MASTER/SIXOSEM_F_STAGE_MASTER_shutdown  Description=SIXOSEMSTAGE_FACE_MASTER
  ISCINF : VIS_LIB/ISCINF
  LogicalOperator : Logic  Operator=NOT  AllPortsSameDT=off  OutDataTypeStr=boolean
  Mux : Mux  Inputs=6
  Mux1 : Mux  Inputs=6
  Mux2 : Mux  Inputs=3
  PAYLOAD : Subsystem
  PAY_DACKILL : cdsDacKill/Subsystem  Description=cdsDacKill
      settings: AttributesFormatString=%<Description>
  PAY_DACKILL_BYPASS_TIME : Constant  Value=0
  PAY_DACKILL_BYPASS_TIMEMON : cdsEpicsOut/Subsystem  Tag=cdsEpicsOutput  Description=|
      | Purpose:                                          
      | Output a FE signal to an EPICS channel.           
      |                                                   
      | Operation:                                        
      | Takes input value and passes it to EPICS record.  
      |                                                   
      | Usage:                                            
      | Name the part with the desired EPICS rrecord name.
      settings: AttributesFormatString=%<Tag>
  PAY_DACKILL_TYPEB : VIS_LIB/DACKILL_TYPEB_PAYLOAD
  PAY_SHUTDOWN : SHUTDOWN/SHUTDOWN
  RO : RelationalOperator  Operator===  OutDataTypeStr=boolean  RndMeth=Nearest
  TM : TM_MASTER/PHASE1_TM_NEW_shutdown
  Terminator{5..6,11..13,15..17,22..23} (10 alike) : Terminator
  IM_V1_OUT : Outport
  IM_V2_OUT : Outport  Port=2
  IM_V3_OUT : Outport  Port=3
  IM_H1_OUT : Outport  Port=4
  IM_H2_OUT : Outport  Port=5
  IM_H3_OUT : Outport  Port=6
  TM_H1_OUT : Outport  Port=7
  TM_H2_Out : Outport  Port=8
  TM_H3_OUT : Outport  Port=9
  TM_H4_OUT : Outport  Port=10
  TM_BIO_CTRL : Outport  Port=11
  IM1_BIO_CTRL : Outport  Port=12
  IM2_BO_CTRL : Outport  Port=13
  CAL_CTRL_OUT : Outport  Port=14
  ISC_IM_OUT : Outport  Port=15
  wires:
  IM/1 -> ISC_IM_OUT/1
  TM/17 -> [TM_OL_DIAGYAW]
  TM/16 -> [TM_OL_DIAGPIT]
  IM/20 -> TM/22
  IM/19 -> TM/21
  CAL_LINE_TM/1 -> TM/19
  CAL_LINE_CTRL/1 -> TM/18
  WD_RESET/1 -> [WD_RESET]
  MASTER_SWITCH/1 -> [MASTERSWITCH]
  BIO_IMH_MON_In/1 -> BIO/6(IMH_MON_In)
  BIO_IMH_ISC_CTRL_In/1 -> BIO/5(IMH_ISC_CTRL)
  BIO/9(IMH_CTRL_Out) -> [IMH_COILOUTF_CTRL]
  BIO/3(TM_CTRL_Out) -> [TM_COILOUTF_CTRL]
  BIO/2(TM_MASK_Out) -> [TM_COILOUTF_MASK]
  BIO/6(IMV_CTRL_Out) -> [IMV_COILOUTF_CTRL]
  BIO/5(IMV_MASK_Out) -> [IMV_COILOUTF_MASK]
  BIO/7(IMH_BO_CTRL_Out) -> IM2_BO_CTRL/1
  BIO/1(TM_BO_CTRL_Out) -> TM_BIO_CTRL/1
  BIO_IMV_MON_In/1 -> BIO/4(IMV_MON_In)
  BIO_IMV_ISC_CTRL_In/1 -> BIO/3(IMV_CTRL)
  BIO_TM_ISC_CTRL_In/1 -> BIO/1(TM_ISC_CTRL)
  BIO/4(IMV_BO_CTRL_Out) -> IM1_BIO_CTRL/1
  BIO_TM_MON_In/1 -> BIO/2(TM_MON_In)
  BIO/8(IMH_MASK_Out) -> [IMH_COILOUTF_MASK]
  [TM_WD] -> PAY_DACKILL_TYPEB/2
  [IM_WD] -> PAY_DACKILL_TYPEB/1
  IM/11 -> Terminator5/1
  TM/9 -> [TM_OL_PIT]
  TM/10 -> [TM_OL_YAW]
  OL_L_Q1/1 -> TM/10
  OL_L_Q2/1 -> TM/11
  OL_L_Q4/1 -> TM/13
  OL_L_Q3/1 -> TM/12
  IM/10 -> [IM_WD]
  TM/5 -> [TM_WD]
  IM/3 -> Terminator13/1
  IM/4 -> IM_V1_OUT/1
  [TM_COILOUTF_MASK] -> TM/5
  [WD_RESET] -> TM/15
  [TM_COILOUTF_CTRL] -> TM/4
  OL_T_Q2/1 -> TM/7
  [MASTERSWITCH] -> TM/14
  OL_T_Q3/1 -> TM/8
  OL_T_Q1/1 -> TM/6
  OL_T_Q4/1 -> TM/9
  TM/8 -> Terminator17/1
  TM/6 -> Terminator15/1
  TM/7 -> Terminator16/1
  IM/2 -> Terminator12/1
  TM/4 -> TM_H4_OUT/1
  TM/2 -> TM_H2_Out/1
  TM/3 -> TM_H3_OUT/1
  TM/1 -> TM_H1_OUT/1
  IM/9 -> IM_H3_OUT/1
  IM/8 -> IM_H2_OUT/1
  IM/7 -> IM_H1_OUT/1
  IM/6 -> IM_V3_OUT/1
  IM/5 -> IM_V2_OUT/1
  IM/12 -> Terminator6/1
  TWR_BLOCKFLAG/1 -> PAY_DACKILL_TYPEB/3
  TM/14 -> CAL_CTRL_OUT/1
  [ShutDown] -> TM/20
  LogicalOperator/1 -> PAY_DACKILL/1
  PAY_DACKILL_BYPASS_TIME/1 -> PAY_DACKILL_BYPASS_TIMEMON/1
  PAY_DACKILL/1 -> Terminator11/1
  PAY_DACKILL_BYPASS_TIMEMON/1 -> PAY_DACKILL/2
  PAY_DACKILL/2 -> Terminator22/1
  PAY_DACKILL_TYPEB/1 -> PAY_SHUTDOWN/1
  PAY_SHUTDOWN/2 -> [ShutState]
  Constant/1 -> RO/1
  [ShutState] -> RO/2
  RO/1 -> Terminator23/1, LogicalOperator/1
  PAY_SHUTDOWN/1 -> [ShutDown]
  IM_OSEM_V1/1 -> IM/1
  IM_OSEM_V2/1 -> IM/2
  IM_OSEM_V3/1 -> IM/3
  IM_OSEM_H1/1 -> IM/4
  IM_OSEM_H2/1 -> IM/5
  IM_OSEM_H3/1 -> IM/6
  Choice/1 -> Mux2/1, IM/7
  Choice1/1 -> Mux2/2, IM/8
  Choice2/1 -> Mux2/3, IM/9
  [ShutDown] -> IM/20
  [TM_OL_YAW] -> IM/19
  [TM_OL_PIT] -> IM/18
  [WD_RESET] -> IM/17
  [MASTERSWITCH] -> IM/16
  [IMH_COILOUTF_MASK] -> IM/15
  [IMV_COILOUTF_MASK] -> IM/13
  [IMH_COILOUTF_CTRL] -> IM/14
  [IMV_COILOUTF_CTRL] -> IM/12
  [DITHER_PIT] -> TM/16
  [DITHER_YAW] -> TM/17
  [DITHER_PIT] -> IM/10
  [DITHER_YAW] -> IM/11
  DITHER_PIT/1 -> [DITHER_PIT]
  DITHER_YAW/1 -> [DITHER_YAW]
  ISC_L/1 -> ISCINF/1
  ISC_P/1 -> ISCINF/2
  ISC_Y/1 -> ISCINF/3
  ISCINF/1 -> Choice/3, TM/1
  ISCINF/2 -> Choice1/3, TM/2
  ISCINF/3 -> Choice2/3, TM/3
  Ground1/1 -> HIER_SWITCH/1
  HIER_SWITCH/1 -> Choice/2, Choice1/2, Choice2/2
  TM/13 -> [TM_LOCK_Y]
  TM/12 -> [TM_LOCK_P]
  TM/11 -> [TM_LOCK_L]
  [TM_LOCK_L] -> Choice/1
  [TM_LOCK_P] -> Choice1/1
  [TM_LOCK_Y] -> Choice2/1
  TM/15 -> [CAS_SW]
  [CAS_SW] -> IM/27
  IM/13 -> Mux/1
  IM/14 -> Mux/2
  IM/15 -> Mux/3
  IM/16 -> Mux/4
  IM/17 -> Mux/5
  IM/18 -> Mux/6
  Mux/1 -> [IM_OSEMOUT]
  Demux/6 -> PAYLOAD/6(IMY_In)
  Demux/5 -> PAYLOAD/5(IMP_In)
  Demux/4 -> PAYLOAD/4(TMR_In)
  Demux/3 -> PAYLOAD/3(IMV_In)
  Demux/2 -> PAYLOAD/2(IMT_In)
  Demux/1 -> PAYLOAD/1(IML_In)
  [IM_OSEMOUT] -> Demux/1
  [TM_OL_DIAGYAW] -> PAYLOAD/8(OLY_In1)
  [TM_OL_DIAGPIT] -> PAYLOAD/7(OLP_In)
  PAYLOAD/1(IML_Out) -> Mux1/1
  PAYLOAD/2(IMT_Out) -> Mux1/2
  PAYLOAD/3(IMV_Out) -> Mux1/3
  PAYLOAD/4(IMR_Out) -> Mux1/4
  PAYLOAD/5(IMP_Out) -> Mux1/5
  PAYLOAD/6(IMY_Out) -> Mux1/6
  Mux1/1 -> [IM_BPACT]
  Demux1/5 -> IM/25
  Demux1/4 -> IM/24
  Demux1/6 -> IM/26
  Demux1/3 -> IM/23
  Demux1/2 -> IM/22
  Demux1/1 -> IM/21
  [IM_BPACT] -> Demux1/1
  Mux2/1 -> [ISC]
  Demux2/1 -> PAYLOAD/9(ISCL_In)
  Demux2/2 -> PAYLOAD/10(ISCP_In)
  Demux2/3 -> PAYLOAD/11(ISCY_In)
  [ISC] -> Demux2/1
